simulink subsystem "TGOV1"  (R2021b)
settings: Solver=VariableStepAuto  StartTime=0.0  StopTime=10.0  RelTol=1e-3
model mask{R=0.05, T_1=0.2, Vmax=1.2, Vmin=0.0, T_2=1, T_3=3, Dt=0}
  mask prompts: R "Permanent droop R (pu)"; T_1 "Steam bowl time constant T_1 (s)"; Vmax "Maximum valve position Vmax (pu)"; Vmin "Minimum valve position Vmin (pu)"; T_2 "Time constant of high-pressure fraction T_2 (s)"; T_3 "Reheater time constant T_3 (s)"; Dt "Turbine damping coefficient Dt (pu)"
libraries: eeGeneralControl x1
settings Model: Creator=ah4430  LastModifiedBy=ah4430

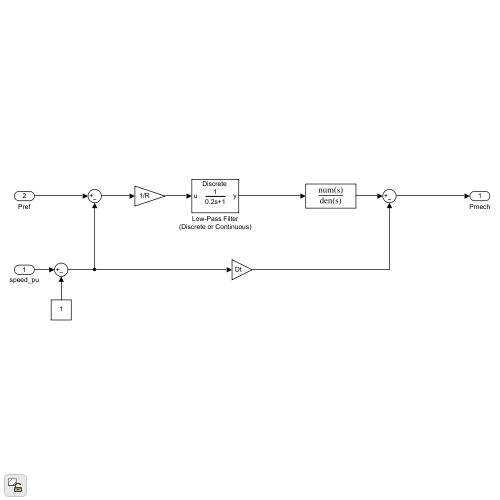
[thumbnail: Simulink's stored preview of the top-level diagram]
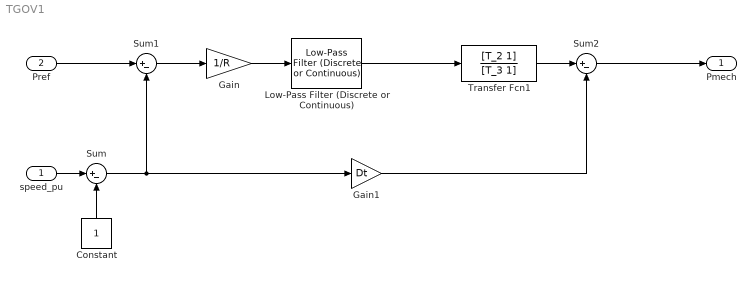
== system TGOV1 ==
  speed_pu : Inport
  Pref : Inport  Port=2
  Constant : Constant
  Gain : Gain  Gain=1/R
  Gain1 : Gain  Gain=Dt
  Low-Pass Filter (Discrete or Continuous) : eeGeneralControl/Low-Pass Filter (Discrete or Continuous)  K=1  T=T_1  B=Vmax  A=Vmin  init_option=Inherited from block input  x0=0  Ts=-1
  Sum : Sum  Inputs=|+-
  Sum1 : Sum  Inputs=|+-
  Sum2 : Sum  Inputs=|+-
  Transfer Fcn1 : TransferFcn  Numerator=[T_2 1]  Denominator=[T_3 1]
  Pmech : Outport
  wires:
  Low-Pass Filter (Discrete or Continuous)/1 -> Transfer Fcn1/1
  Constant/1 -> Sum/2
  Gain1/1 -> Sum2/2
  Sum/1 -> Sum1/2, Gain1/1
  Sum1/1 -> Gain/1
  Pref/1 -> Sum1/1
  Transfer Fcn1/1 -> Sum2/1
  Sum2/1 -> Pmech/1
  speed_pu/1 -> Sum/1
  Gain/1 -> Low-Pass Filter (Discrete or Continuous)/1
